simulink model "A29_npc_threelevel_new"  (R2017a)
settings: Solver=ode4  StartTime=0.0  StopTime=0.04  FixedStep=1e-6  MaxStep=1e-4  RelTol=1e-3
InitFcn:
  | v=3000
  | r=0.000001
  | c=1000e-6
  | l=314
  | i=1000
  | r1=1000
  | t=1/3000
  | ma=2
  | f=2*pi*50
  | p1=(2*pi)/3
  | p2=-(2*pi)/3
libraries: powerlib x36, simulink x6
settings Model: Creator=dell  LastModifiedBy=A_M

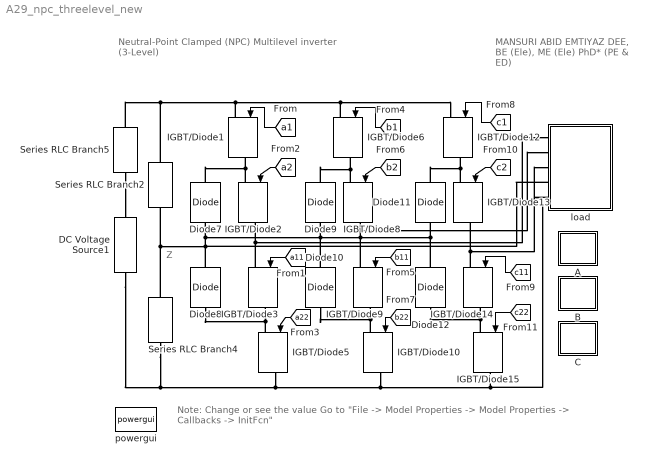
== system A29_npc_threelevel_new ==
  note: Z
  note: Neutral-Point Clamped (NPC)
      | Multilevel inverter (3-Level)
  note: Note: Change or see the value
      | Go to "File -> Model Properties -> Model Properties -> Callbacks -> InitFcn"
  note: MANSURI ABID EMTIYAZ
      | DEE, BE (Ele), ME (Ele)
      | PhD* (PE & ED)
  A : Subsystem
  B : Subsystem
  C : Subsystem
  DC Voltage Source1 : powerlib/Electrical Sources/DC Voltage Source  Amplitude=v  Measurements=None
  Diode{7..12} (6 alike) : powerlib/Power Electronics/Diode  Ron=0.001  Lon=0  Vf=0.8  IC=0  UseSnubber=0  Rs=500  Cs=250e-9  Measurements=off
  IGBT/Diode{1..3,5..6,8..10,12..15} (12 alike) : powerlib/Power Electronics/IGBT//Diode  Ron=1e-3  Rs=1e5  Cs=inf  Measurements=off
  Series RLC Branch2 : powerlib/Elements/Series RLC Branch  LConnTagsString=__new0  RConnTagsString=__new0  BranchType=C  Resistance=1  Inductance=1e-3  SetiL0=off  InitialCurrent=0  Capacitance=c  Setx0=on  InitialVoltage=i  Measurements=None
  Series RLC Branch4 : powerlib/Elements/Series RLC Branch  LConnTagsString=__new0  RConnTagsString=__new0  BranchType=C  Resistance=1  Inductance=1e-3  SetiL0=off  InitialCurrent=0  Capacitance=c  Setx0=on  InitialVoltage=i  Measurements=None
  Series RLC Branch5 : powerlib/Elements/Series RLC Branch  LConnTagsString=__new0  RConnTagsString=__new0  BranchType=R  Resistance=r  Inductance=1e-3  SetiL0=off  InitialCurrent=0  Capacitance=1e-6  Setx0=off  InitialVoltage=0  Measurements=None
  load : Subsystem
  powergui : powerlib/powergui  Priority=1  SimulationMode=Discrete  SampleTime=1e-6  frequency=60  Iterations=50  frequencyindice=0  Pbase=100e6  ErrMax=1e-4  UnitsV=kV  UnitsW=MW  buscounter=0  FunctionMessages=off  echomessages=off  EnableUseOfTLC=off  CurrentSourceSwitches=off  DisableSnubberDevices=off  DisableRonSwitches=off  DisableVfSwitches=off  DisplayEquations=off  SolverType=Tustin/Backward Euler (TBE)  Interpol=off  ExternalGateDelay=off  methode=off  Ts=100  x0status=blocks  SPID=on  SwTol=0  HookPort=off  RestoreLinks=warning  ResistiveCurrentMeasurement=off  Frange=[0:2:500]  Ylog=off  Xlog=on  ShowGrid=off  save=off  variable=ZData  structure=d  ZoomFFT=off  StartTime=0.2  cycles=2  DisplayStyle=1  fundamental=50  FreqAxis=on  MaxFrequency=40000  frequencyindicesteady=1  RmsSteady=1  display=off
  wires:
  [a1] -> IGBT/Diode1/1
  [a2] -> IGBT/Diode2/1
  [a11] -> IGBT/Diode3/1
  [a22] -> IGBT/Diode5/1
  [b1] -> IGBT/Diode6/1
  [b2] -> IGBT/Diode8/1
  [b11] -> IGBT/Diode9/1
  [b22] -> IGBT/Diode10/1
  [c11] -> IGBT/Diode14/1
  [c1] -> IGBT/Diode12/1
  [c2] -> IGBT/Diode13/1
  [c22] -> IGBT/Diode15/1
  connections:
  IGBT/Diode2/LConn1 -- Diode7/RConn1 -- IGBT/Diode1/RConn1
  IGBT/Diode3/LConn1 -- load/LConn1 -- IGBT/Diode2/RConn1
  IGBT/Diode5/LConn1 -- Diode8/LConn1 -- IGBT/Diode3/RConn1
  IGBT/Diode8/LConn1 -- Diode9/RConn1 -- IGBT/Diode6/RConn1
  IGBT/Diode9/LConn1 -- IGBT/Diode8/RConn1 -- load/LConn2
  IGBT/Diode10/LConn1 -- Diode10/LConn1 -- IGBT/Diode9/RConn1
  IGBT/Diode13/LConn1 -- Diode11/RConn1 -- IGBT/Diode12/RConn1
  IGBT/Diode14/LConn1 -- load/LConn3 -- IGBT/Diode13/RConn1
  IGBT/Diode15/LConn1 -- Diode12/LConn1 -- IGBT/Diode14/RConn1
  Series RLC Branch4/LConn1 -- load/LConn4 -- Diode12/RConn1 -- Diode11/LConn1 -- Diode10/RConn1 -- Diode9/LConn1 -- Diode7/LConn1 -- Diode8/RConn1 -- Series RLC Branch2/RConn1
  Series RLC Branch5/LConn1 -- DC Voltage Source1/RConn1
  Series RLC Branch5/RConn1 -- Series RLC Branch2/LConn1 -- IGBT/Diode1/LConn1 -- IGBT/Diode6/LConn1 -- IGBT/Diode12/LConn1
  DC Voltage Source1/LConn1 -- Series RLC Branch4/RConn1 -- IGBT/Diode5/RConn1 -- IGBT/Diode10/RConn1 -- load/LConn5 -- IGBT/Diode15/RConn1

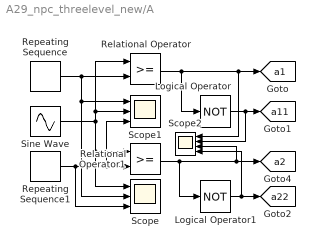
== system A29_npc_threelevel_new/A ==
  Logical Operator : Logic  Operator=NOT  AllPortsSameDT=off  OutDataTypeStr=boolean
  Logical Operator1 : Logic  Operator=NOT  AllPortsSameDT=off  OutDataTypeStr=boolean
  Relational Operator : RelationalOperator  OutDataTypeStr=boolean  RndMeth=Simplest
  Relational Operator1 : RelationalOperator  OutDataTypeStr=boolean  RndMeth=Simplest
  Repeating Sequence : simulink/Sources/Repeating Sequence  rep_seq_t=[0 t/2 t]  rep_seq_y=[0 2 0]
  Repeating Sequence1 : simulink/Sources/Repeating Sequence  rep_seq_t=[0 t/2 t]  rep_seq_y=[-2 0 -2]
  Scope : Scope  NumInputPorts=3
  Scope1 : Scope  NumInputPorts=3
  Scope2 : Scope  NumInputPorts=4
  Sine Wave : Sin  Amplitude=ma  Frequency=f  SampleTime=0
  tag scope: a11=global, a1=global, a22=global, a2=global
  wires:
  Logical Operator/1 -> Scope2/2, [a11]
  Logical Operator1/1 -> [a22], Scope2/4
  Repeating Sequence/1 -> Scope1/1, Scope/2, Relational Operator/2
  Repeating Sequence1/1 -> Scope/3, Scope1/3, Relational Operator1/2
  Relational Operator/1 -> Scope2/1, [a1], Logical Operator/1
  Relational Operator1/1 -> Logical Operator1/1, Scope2/3, [a2]
  Sine Wave/1 -> Scope/1, Relational Operator1/1, Scope1/2, Relational Operator/1

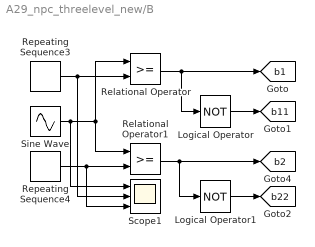
== system A29_npc_threelevel_new/B ==
  Logical Operator : Logic  Operator=NOT  AllPortsSameDT=off  OutDataTypeStr=boolean
  Logical Operator1 : Logic  Operator=NOT  AllPortsSameDT=off  OutDataTypeStr=boolean
  Relational Operator : RelationalOperator  OutDataTypeStr=boolean  RndMeth=Simplest
  Relational Operator1 : RelationalOperator  OutDataTypeStr=boolean  RndMeth=Simplest
  Repeating Sequence3 : simulink/Sources/Repeating Sequence  rep_seq_t=[0 t/2 t]  rep_seq_y=[0 2 0]
  Repeating Sequence4 : simulink/Sources/Repeating Sequence  rep_seq_t=[0 t/2 t]  rep_seq_y=[-2 0 -2]
  Scope1 : Scope  NumInputPorts=3
  Sine Wave : Sin  Amplitude=ma  Frequency=f  Phase=p2  SampleTime=0
  tag scope: b11=global, b1=global, b22=global, b2=global
  wires:
  Logical Operator1/1 -> [b22]
  Repeating Sequence3/1 -> Scope1/2, Relational Operator/2
  Repeating Sequence4/1 -> Scope1/3, Relational Operator1/2
  Sine Wave/1 -> Scope1/1, Relational Operator1/1, Relational Operator/1
  Relational Operator1/1 -> Logical Operator1/1, [b2]
  Relational Operator/1 -> Logical Operator/1, [b1]
  Logical Operator/1 -> [b11]

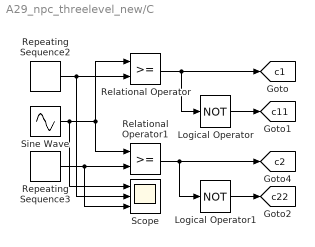
== system A29_npc_threelevel_new/C ==
  Logical Operator : Logic  Operator=NOT  AllPortsSameDT=off  OutDataTypeStr=boolean
  Logical Operator1 : Logic  Operator=NOT  AllPortsSameDT=off  OutDataTypeStr=boolean
  Relational Operator : RelationalOperator  OutDataTypeStr=boolean  RndMeth=Simplest
  Relational Operator1 : RelationalOperator  OutDataTypeStr=boolean  RndMeth=Simplest
  Repeating Sequence2 : simulink/Sources/Repeating Sequence  rep_seq_t=[0 t/2 t]  rep_seq_y=[0 2 0]
  Repeating Sequence3 : simulink/Sources/Repeating Sequence  rep_seq_t=[0 t/2 t]  rep_seq_y=[-2 0 -2]
  Scope : Scope  NumInputPorts=3
  Sine Wave : Sin  Amplitude=ma  Frequency=f  Phase=p1  SampleTime=0
  tag scope: c11=global, c1=global, c22=global, c2=global
  wires:
  Logical Operator1/1 -> [c22]
  Repeating Sequence2/1 -> Scope/2, Relational Operator/2
  Repeating Sequence3/1 -> Scope/3, Relational Operator1/2
  Sine Wave/1 -> Scope/1, Relational Operator1/1, Relational Operator/1
  Relational Operator1/1 -> Logical Operator1/1, [c2]
  Relational Operator/1 -> Logical Operator/1, [c1]
  Logical Operator/1 -> [c11]

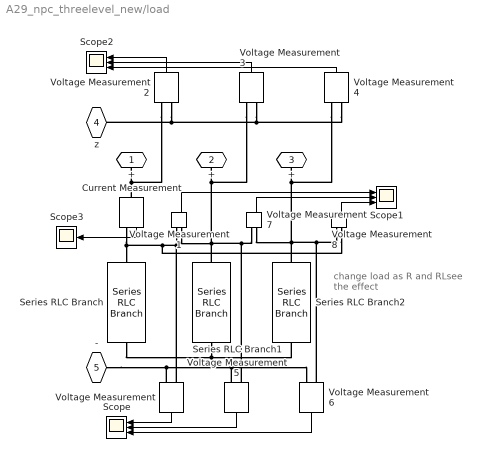
== system A29_npc_threelevel_new/load ==
  note: change load as R and RLsee the effect
  Current Measurement : powerlib/Measurements/Current Measurement  PhasorSimulation=off  OutputType=Complex  PSBequivalent=0
  Scope : Scope  NumInputPorts=3
  Scope1 : Scope  NumInputPorts=3
  Scope2 : Scope  NumInputPorts=3
  Scope3 : Scope
  Series RLC Branch : powerlib/Elements/Series RLC Branch  LConnTagsString=__new0  RConnTagsString=__new0  BranchType=R  Resistance=r1  Inductance=l  SetiL0=off  InitialCurrent=0  Capacitance=1e-6  Setx0=off  InitialVoltage=0  Measurements=None
  Series RLC Branch1 : powerlib/Elements/Series RLC Branch  LConnTagsString=__new0  RConnTagsString=__new0  BranchType=R  Resistance=r1  Inductance=l  SetiL0=off  InitialCurrent=0  Capacitance=1e-6  Setx0=off  InitialVoltage=0  Measurements=None
  Series RLC Branch2 : powerlib/Elements/Series RLC Branch  LConnTagsString=__new0  RConnTagsString=__new0  BranchType=R  Resistance=r1  Inductance=l  SetiL0=off  InitialCurrent=0  Capacitance=1e-6  Setx0=off  InitialVoltage=0  Measurements=None
  Voltage Measurement{,1..8} (9 alike) : powerlib/Measurements/Voltage Measurement  PhasorSimulation=off  OutputType=Complex  PSBequivalent=0
  + : PMIOPort  Port=1  Side=Left
  "+  " : PMIOPort  Port=2  Side=Left
  "+   " : PMIOPort  Port=3  Side=Left
  z : PMIOPort  Port=4  Side=Left
  - : PMIOPort  Port=5  Side=Left
  wires:
  Current Measurement/1 -> Scope3/1
  Voltage Measurement/1 -> Scope/1
  Voltage Measurement5/1 -> Scope/2
  Voltage Measurement6/1 -> Scope/3
  Voltage Measurement1/1 -> Scope1/1
  Voltage Measurement7/1 -> Scope1/2
  Voltage Measurement8/1 -> Scope1/3
  Voltage Measurement2/1 -> Scope2/1
  Voltage Measurement3/1 -> Scope2/2
  Voltage Measurement4/1 -> Scope2/3
  connections:
  "+   "/RConn1 -- Series RLC Branch2/LConn1 -- Voltage Measurement8/LConn1 -- Voltage Measurement6/LConn1 -- Voltage Measurement7/LConn2 -- Voltage Measurement4/LConn1
  "+  "/RConn1 -- Series RLC Branch1/LConn1 -- Voltage Measurement7/LConn1 -- Voltage Measurement5/LConn1 -- Voltage Measurement1/LConn2 -- Voltage Measurement3/LConn1
  Series RLC Branch/RConn1 -- Series RLC Branch2/RConn1 -- Series RLC Branch1/RConn1
  Current Measurement/RConn1 -- Voltage Measurement8/LConn2 -- Voltage Measurement1/LConn1 -- Voltage Measurement/LConn1 -- Series RLC Branch/LConn1
  +/RConn1 -- Current Measurement/LConn1 -- Voltage Measurement2/LConn1
  Voltage Measurement2/LConn2 -- Voltage Measurement4/LConn2 -- Voltage Measurement3/LConn2 -- z/RConn1
  -/RConn1 -- Voltage Measurement/LConn2 -- Voltage Measurement5/LConn2 -- Voltage Measurement6/LConn2
